simulink model "motor_cc_simu"  (R2024a)
settings: Solver=VariableStepAuto  StartTime=0.0  StopTime=10.0  RelTol=1e-3
values from neighbouring files (symbols this model uses):
  K = 0.75    [motor_cc.mat]
  T = 0.4    [motor_cc.mat]
settings Model: Creator=18.01775-4  LastModifiedBy=18.01775-4

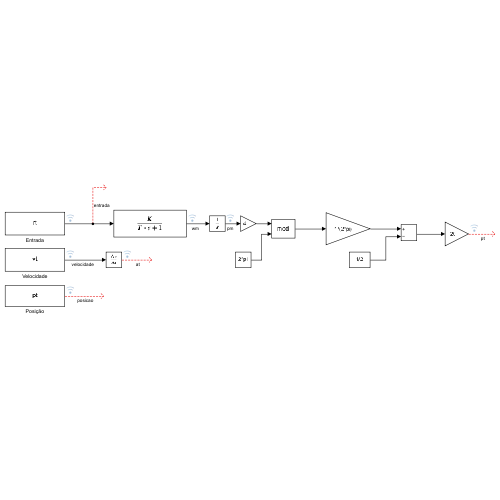
[thumbnail: Simulink's stored preview of the top-level diagram]
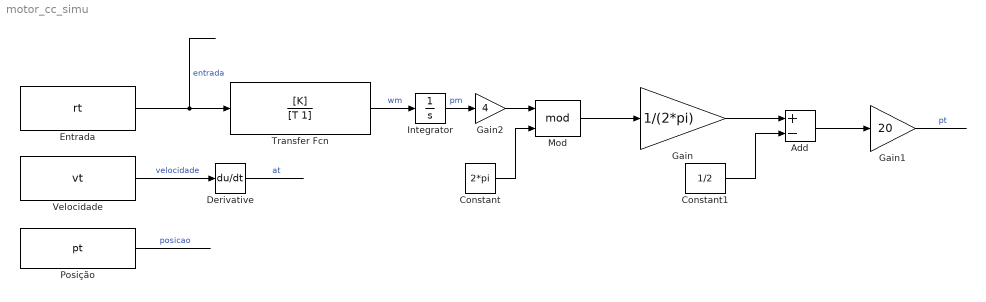
== system motor_cc_simu ==
  Add : Sum  Inputs=+-
  Constant : Constant  Value=2*pi
  Constant1 : Constant  Value=1/2
  Derivative : Derivative
  Entrada : FromWorkspace  VariableName=rt  SampleTime=0.01
  Gain : Gain  Gain=1/(2*pi)
  Gain1 : Gain  Gain=20
  Gain2 : Gain  Gain=4
  Integrator : Integrator
  Mod : Math  Operator=mod
  Posição : FromWorkspace  VariableName=pt  SampleTime=0.01
  Transfer Fcn : TransferFcn  Numerator=[K]  Denominator=[T 1]
  Velocidade : FromWorkspace  VariableName=vt  SampleTime=0.01
  wires:
  Velocidade/1 -> Derivative/1  "velocidade"
  Posição/1 -> ?  "posicao"
  Transfer Fcn/1 -> Integrator/1  "wm"
  Entrada/1 -> Transfer Fcn/1  "entrada"
  Integrator/1 -> Gain2/1  "pm"
  Derivative/1 -> ?  "at"
  Constant/1 -> Mod/2
  Mod/1 -> Gain/1
  Constant1/1 -> Add/2
  Gain/1 -> Add/1
  Add/1 -> Gain1/1
  Gain1/1 -> ?  "pt"
  Gain2/1 -> Mod/1
